simulink model "third"  (R2023a)
settings: Solver=FixedStepAuto  StartTime=0.0  StopTime=10  FixedStep=0.01  RelTol=1e-3
libraries: simulink x2
settings Model: Creator=evdokiiagalkina  LastModifiedBy=evdokiiagalkina

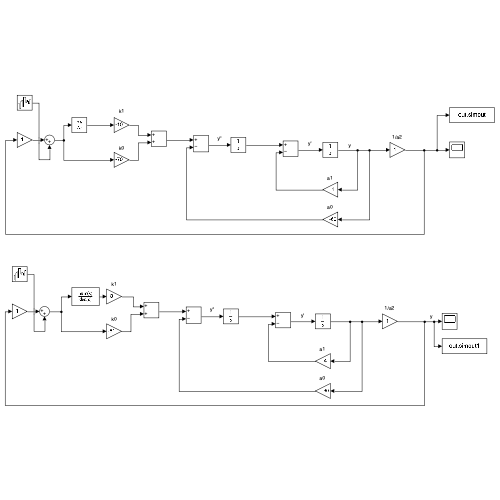
[thumbnail: Simulink's stored preview of the top-level diagram]
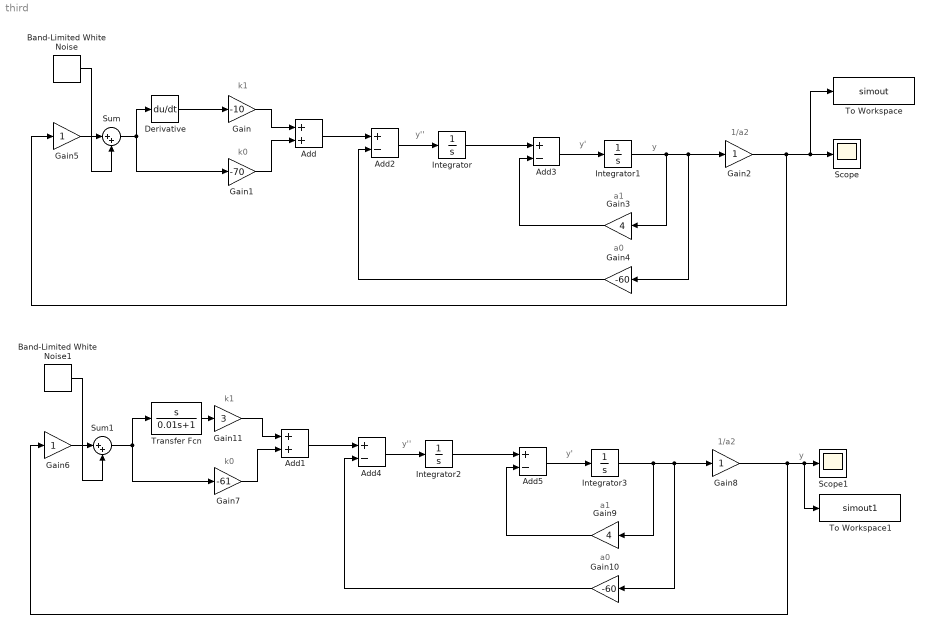
== system third ==
  note: k1
  note: 1/a2
  note: a0
  note: k0
  note: k1
  note: y'
  note: a1
  note: y''
  note: y
  note: y
  note: k0
  note: a0
  note: y'
  note: a1
  note: 1/a2
  note: y''
  Add : Sum
  Add1 : Sum
  Add{2..5} (4 alike) : Sum  Inputs=+-
  Band-Limited White Noise : simulink/Sources/Band-Limited White Noise  Cov=[0.01]  Ts=0.01  seed=[23341]
  Band-Limited White Noise1 : simulink/Sources/Band-Limited White Noise  Cov=[0.01]  Ts=0.01  seed=[23341]
  Derivative : Derivative
  Gain : Gain  Gain=-10
  Gain1 : Gain  Gain=-70
  Gain10 : Gain  Gain=-60
  Gain11 : Gain  Gain=3
  Gain{2,5..6,8} (4 alike) : Gain
  Gain3 : Gain  Gain=4
  Gain4 : Gain  Gain=-60
  Gain7 : Gain  Gain=-61
  Gain9 : Gain  Gain=4
  Integrator{,1..3} (4 alike) : Integrator  InitialCondition=5
  Scope : Scope
  Scope1 : Scope
  Sum : Sum  Inputs=|++
  Sum1 : Sum  Inputs=|++
  To Workspace : ToWorkspace  VariableName=simout  SaveFormat=Timeseries  SampleTime=-1
  To Workspace1 : ToWorkspace  VariableName=simout1  SaveFormat=Timeseries  SampleTime=-1
  Transfer Fcn : TransferFcn  Numerator=[1 0]  Denominator=[0.01 1]
  wires:
  Gain2/1 -> Gain5/1, To Workspace/1, Scope/1
  Gain1/1 -> Add/2
  Gain3/1 -> Add3/2
  Integrator/1 -> Add3/1
  Add2/1 -> Integrator/1
  Add/1 -> Add2/1
  Integrator1/1 -> Gain3/1, Gain4/1, Gain2/1
  Gain4/1 -> Add2/2
  Add3/1 -> Integrator1/1
  Derivative/1 -> Gain/1
  Gain/1 -> Add/1
  Add4/1 -> Integrator2/1
  Add1/1 -> Add4/1
  Gain10/1 -> Add4/2
  Gain7/1 -> Add1/2
  Add5/1 -> Integrator3/1
  Gain9/1 -> Add5/2
  Integrator2/1 -> Add5/1
  Gain8/1 -> Gain6/1, To Workspace1/1, Scope1/1
  Integrator3/1 -> Gain9/1, Gain10/1, Gain8/1
  Gain5/1 -> Sum/1
  Band-Limited White Noise/1 -> Sum/2
  Sum/1 -> Gain1/1, Derivative/1
  Band-Limited White Noise1/1 -> Sum1/2
  Gain6/1 -> Sum1/1
  Sum1/1 -> Gain7/1, Transfer Fcn/1
  Transfer Fcn/1 -> Gain11/1
  Gain11/1 -> Add1/1
